simulink library "INT_EnvP_VD"  (R2016b)
settings: Solver=VariableStepAuto  StartTime=0.0  StopTime=10.0  RelTol=1e-3
settings Model: Creator=Administrator  LastModifiedBy=Administrator

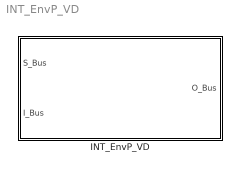
== system INT_EnvP_VD ==
  INT_EnvP_VD : Subsystem

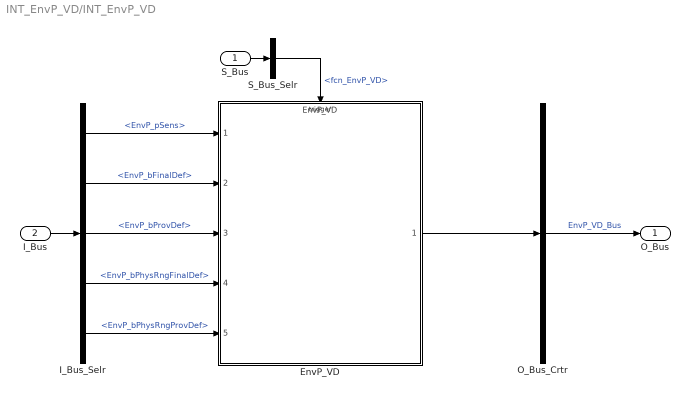
== system INT_EnvP_VD/INT_EnvP_VD ==
  S_Bus : Inport
  I_Bus : Inport  Port=2
  EnvP_VD : ModelReference  ModelNameDialog=EnvP_VD  SimulationMode=Normal  ModelReferenceVersion=1.7  TriggerPortName=function  TriggerPortTriggerType=function-call  TriggerPortStatesWhenEnabling=held
  I_Bus_Selr : BusSelector  OutputSignals=EnvP_pSens,EnvP_bFinalDef,EnvP_bProvDef,EnvP_bPhysRngFinalDef,EnvP_bPhysRngProvDef
  O_Bus_Crtr : BusCreator  Inputs=1
  S_Bus_Selr : BusSelector  OutputSignals=fcn_EnvP_VD
  O_Bus : Outport
  wires:
  S_Bus_Selr/1 -> EnvP_VD/Trigger  "<fcn_EnvP_VD>"
  S_Bus/1 -> S_Bus_Selr/1
  I_Bus/1 -> I_Bus_Selr/1
  I_Bus_Selr/1 -> EnvP_VD/1  "<EnvP_pSens>"
  I_Bus_Selr/2 -> EnvP_VD/2  "<EnvP_bFinalDef>"
  I_Bus_Selr/3 -> EnvP_VD/3  "<EnvP_bProvDef>"
  I_Bus_Selr/4 -> EnvP_VD/4  "<EnvP_bPhysRngFinalDef>"
  I_Bus_Selr/5 -> EnvP_VD/5  "<EnvP_bPhysRngProvDef>"
  O_Bus_Crtr/1 -> O_Bus/1  "EnvP_VD_Bus"
  EnvP_VD/1 -> O_Bus_Crtr/1
